simulink library "switchboard"  (R2013a)
settings: Solver=ode3  StartTime=0.0  StopTime=10.0  RelTol=1e-3
libraries: switchboard x2, goto x1
settings Model: Creator=torstebo  LastModifiedBy=torstebo

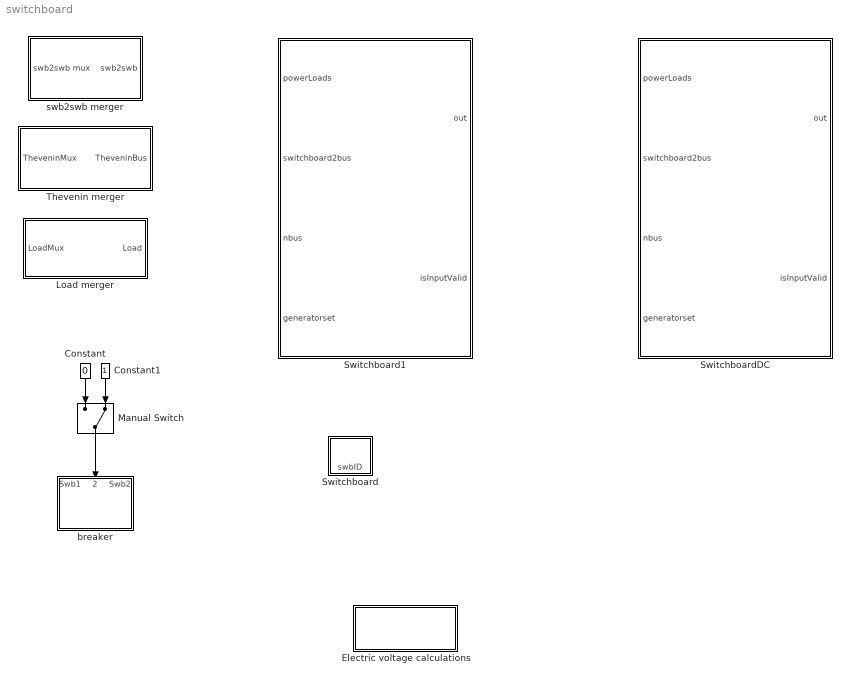
== system switchboard ==
  Constant : Constant  Value=0  OutDataTypeStr=boolean
  Constant1 : Constant  OutDataTypeStr=boolean
  Electric voltage calculations : Subsystem
  Load merger : Subsystem
  Manual Switch : ManualSwitch  CurrentSetting=0
  Switchboard : Subsystem  Tag=Switchboard  mask{swbId=0}
      mask prompts: swbId "Switchboard ID"
  Switchboard1 : MATLAB Function  TreatAsAtomicUnit=on
  SwitchboardDC : MATLAB Function  TreatAsAtomicUnit=on
  Thevenin merger : Subsystem
  breaker : Subsystem  Tag=SwitchboardBreaker  mask{id=0}
  swb2swb merger : Subsystem
  wires:
  Constant/1 -> Manual Switch/1
  Constant1/1 -> Manual Switch/2
  Manual Switch/1 -> breaker/2(Breaker)

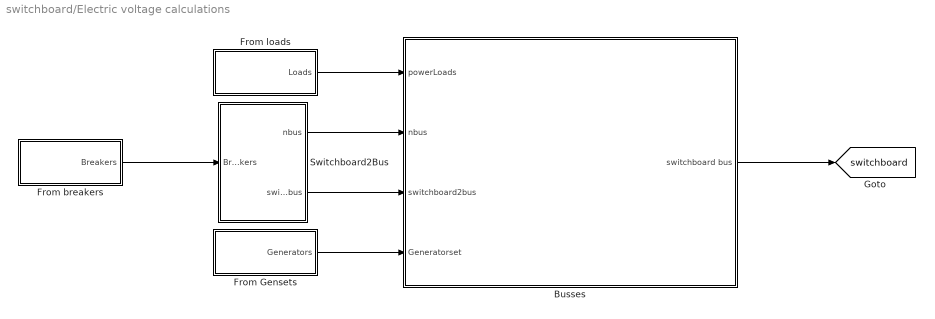
== system switchboard/Electric voltage calculations ==
  Busses : Subsystem
      mask Display:
      | image(imread('figs/switchboard.jpg'))
      | port_label('input',1,'Power Loads')
      | port_label('input',2,'nbus')
      | port_label('input',3,'switchboard2bus')
      | port_label('input',4,'Generators')
      | port_label('output',1,'switchboard')
  From Gensets : Subsystem  Tag=FromGeneratorsetElectric
  From breakers : Subsystem  Tag=FromBreakers
  From loads : Subsystem  Tag=FromLoads
  Switchboard2Bus : Subsystem  Tag=Switchboard2Bus  mask{nSwitchboards=3}
      mask prompts: nSwitchboards "Number of Switchboards"
  tag scope: switchboard=global
  wires:
  From breakers/1(Breakers) -> Switchboard2Bus/1(Breakers)
  From loads/1(Loads) -> Busses/1(powerLoads)
  From Gensets/1(Generators) -> Busses/4(Generatorset)
  Switchboard2Bus/2(switchboard2bus) -> Busses/3(switchboard2bus)
  Switchboard2Bus/1(nbus) -> Busses/2(nbus)
  Busses/1(switchboard bus) -> [switchboard]

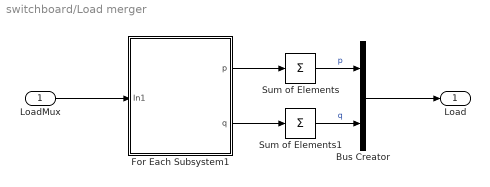
== system switchboard/Load merger ==
  LoadMux : Inport
  Bus Creator : BusCreator  Inputs='p','q'  OutDataTypeStr=Bus: powerLoadsBus  NonVirtualBus=on
  For Each Subsystem1 : Subsystem  TreatAsAtomicUnit=on
  Sum of Elements : Sum  Inputs=+
  Sum of Elements1 : Sum  Inputs=+
  Load : Outport  OutDataTypeStr=Bus: powerLoadsBus
  wires:
  For Each Subsystem1/2(q) -> Sum of Elements1/1
  Sum of Elements1/1 -> Bus Creator/2  "q"
  Sum of Elements/1 -> Bus Creator/1  "p"
  For Each Subsystem1/1(p) -> Sum of Elements/1
  Bus Creator/1 -> Load/1
  LoadMux/1 -> For Each Subsystem1/1(In1)

== system switchboard/Switchboard ==
  Switchboard : Constant  Value=swbId
  swbID : Outport
  wires:
  Switchboard/1 -> swbID/1

== system switchboard/Thevenin merger ==
  TheveninMux : Inport
  For Each Subsystem : Subsystem  TreatAsAtomicUnit=on
  MATLAB Function : MATLAB Function  TreatAsAtomicUnit=on
  TheveninBus : Outport  OutDataTypeStr=Bus: TheveninBus
  wires:
  For Each Subsystem/5(omega) -> MATLAB Function/5(omega)
  For Each Subsystem/2(z) -> MATLAB Function/2(z)
  For Each Subsystem/1(e) -> MATLAB Function/1(e)
  TheveninMux/1 -> For Each Subsystem/1(In1)
  For Each Subsystem/4(Connected) -> MATLAB Function/4(on)
  MATLAB Function/1(thevenin_bus) -> TheveninBus/1
  For Each Subsystem/3(Sb) -> MATLAB Function/3(Sb)

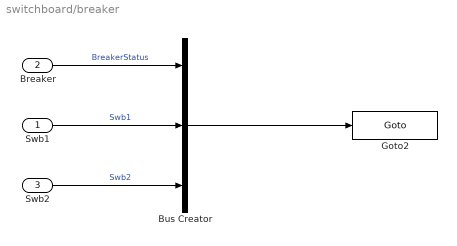
== system switchboard/breaker ==
  Swb1 : Inport
  Breaker : Inport  Port=2
  Swb2 : Inport  Port=3
  Bus Creator : BusCreator  Inputs=3  OutDataTypeStr=Bus: Breaker  NonVirtualBus=on
  Goto2 : goto/Goto  GotoTag=sprintf('Breaker%d',id)
  wires:
  Swb1/1 -> Bus Creator/2  "Swb1"
  Breaker/1 -> Bus Creator/1  "BreakerStatus"
  Swb2/1 -> Bus Creator/3  "Swb2"
  Bus Creator/1 -> Goto2/1

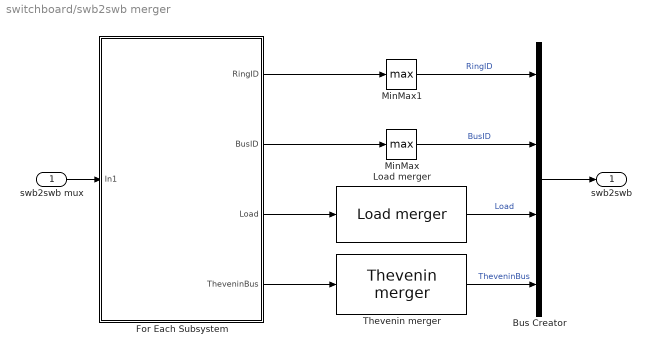
== system switchboard/swb2swb merger ==
  swb2swb mux : Inport
  Bus Creator : BusCreator  Inputs='RingID','BusID','Load','TheveninBus'  OutDataTypeStr=Bus: swb2swb  NonVirtualBus=on
  For Each Subsystem : Subsystem  TreatAsAtomicUnit=on
  Load merger : switchboard/Load merger
  MinMax : MinMax  Function=max
  MinMax1 : MinMax  Function=max
  Thevenin merger : switchboard/Thevenin merger
  swb2swb : Outport  OutDataTypeStr=Bus: swb2swb
  wires:
  For Each Subsystem/1(RingID) -> MinMax1/1
  MinMax1/1 -> Bus Creator/1  "RingID"
  MinMax/1 -> Bus Creator/2  "BusID"
  Thevenin merger/1 -> Bus Creator/4  "TheveninBus"
  Load merger/1 -> Bus Creator/3  "Load"
  For Each Subsystem/2(BusID) -> MinMax/1
  For Each Subsystem/3(Load) -> Load merger/1
  For Each Subsystem/4(TheveninBus) -> Thevenin merger/1
  swb2swb mux/1 -> For Each Subsystem/1(In1)
  Bus Creator/1 -> swb2swb/1

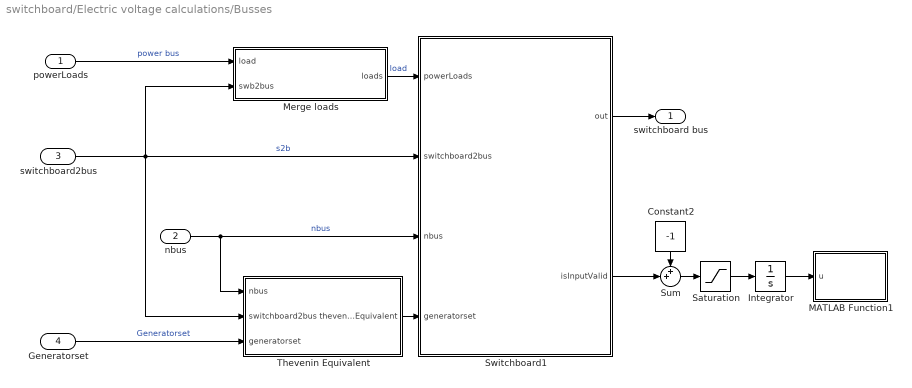
== system switchboard/Electric voltage calculations/Busses ==
  powerLoads : Inport  OutDataTypeStr=Bus: powerLoadsBus
  nbus : Inport  Port=2
  switchboard2bus : Inport  Port=3
  Generatorset : Inport  Port=4
  Constant2 : Constant  Value=-1
  Integrator : Integrator
  MATLAB Function1 : MATLAB Function  TreatAsAtomicUnit=on
  Merge loads : MATLAB Function  TreatAsAtomicUnit=on
  Saturation : Saturate  UpperLimit=0  LowerLimit=-1
  Sum : Sum  Inputs=++|
  Switchboard1 : MATLAB Function  TreatAsAtomicUnit=on
  Thevenin Equivalent : MATLAB Function  TreatAsAtomicUnit=on
  switchboard bus : Outport
  wires:
  Switchboard1/1(out) -> switchboard bus/1
  powerLoads/1 -> Merge loads/1(load)  "power bus"
  switchboard2bus/1 -> Switchboard1/2(switchboard2bus), Merge loads/2(swb2bus), Thevenin Equivalent/2(switchboard2bus)  "s2b"
  Generatorset/1 -> Thevenin Equivalent/3(generatorset)  "Generatorset"
  Integrator/1 -> MATLAB Function1/1(u)
  Constant2/1 -> Sum/1
  Sum/1 -> Saturation/1
  Switchboard1/2(isInputValid) -> Sum/2
  nbus/1 -> Switchboard1/3(nbus), Thevenin Equivalent/1(nbus)  "nbus"
  Merge loads/1(loads) -> Switchboard1/1(powerLoads)  "load"
  Thevenin Equivalent/1(theveninEquivalent) -> Switchboard1/4(generatorset)
  Saturation/1 -> Integrator/1

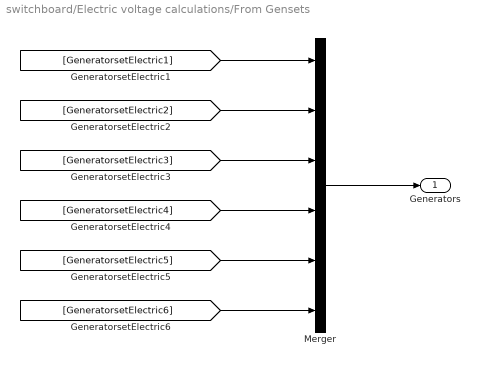
== system switchboard/Electric voltage calculations/From Gensets ==
  Merger : Concatenate  Tag=FromGeneratorsetElectric/Merger  NumInputs=6
  Generators : Outport
  wires:
  Merger/1 -> Generators/1
  [GeneratorsetElectric1] -> Merger/1
  [GeneratorsetElectric2] -> Merger/2
  [GeneratorsetElectric6] -> Merger/6
  [GeneratorsetElectric3] -> Merger/3
  [GeneratorsetElectric4] -> Merger/4
  [GeneratorsetElectric5] -> Merger/5

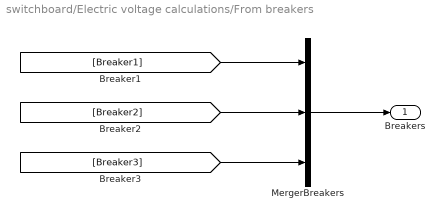
== system switchboard/Electric voltage calculations/From breakers ==
  MergerBreakers : Concatenate  Tag=FromBreakers/MergerBreakers  NumInputs=3
  Breakers : Outport
  wires:
  MergerBreakers/1 -> Breakers/1
  [Breaker1] -> MergerBreakers/1
  [Breaker2] -> MergerBreakers/2
  [Breaker3] -> MergerBreakers/3

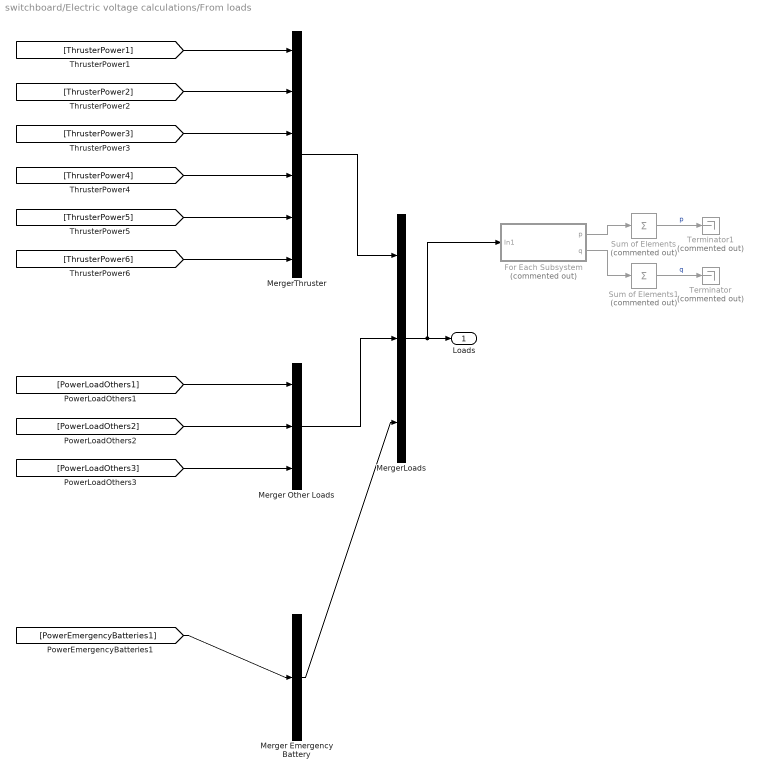
== system switchboard/Electric voltage calculations/From loads ==
  For Each Subsystem : Subsystem  Commented=on  TreatAsAtomicUnit=on
  Merger Emergency Battery : Concatenate  Tag=FromLoads/MergerEmergencyBattery  NumInputs=1
  Merger Other Loads : Concatenate  Tag=FromLoads/MergerOtherLoads  NumInputs=3
  MergerLoads : Concatenate  Tag=FromLoads/MergerLoads  NumInputs=3
  MergerThruster : Concatenate  Tag=FromLoads/MergerThruster  NumInputs=6
  Sum of Elements : Sum  Commented=on  Inputs=+
  Sum of Elements1 : Sum  Commented=on  Inputs=+
  Terminator : Terminator  Commented=on
  Terminator1 : Terminator  Commented=on
  Loads : Outport
  wires:
  MergerThruster/1 -> MergerLoads/1
  Merger Other Loads/1 -> MergerLoads/2
  MergerLoads/1 -> For Each Subsystem/1(In1), Loads/1
  For Each Subsystem/1(p) -> Sum of Elements/1
  For Each Subsystem/2(q) -> Sum of Elements1/1
  Sum of Elements1/1 -> Terminator/1  "q"
  Sum of Elements/1 -> Terminator1/1  "p"
  Merger Emergency Battery/1 -> MergerLoads/3
  [PowerLoadOthers1] -> Merger Other Loads/1
  [PowerLoadOthers2] -> Merger Other Loads/2
  [PowerLoadOthers3] -> Merger Other Loads/3
  [ThrusterPower1] -> MergerThruster/1
  [ThrusterPower2] -> MergerThruster/2
  [ThrusterPower3] -> MergerThruster/3
  [ThrusterPower4] -> MergerThruster/4
  [ThrusterPower5] -> MergerThruster/5
  [ThrusterPower6] -> MergerThruster/6
  [PowerEmergencyBatteries1] -> Merger Emergency Battery/1

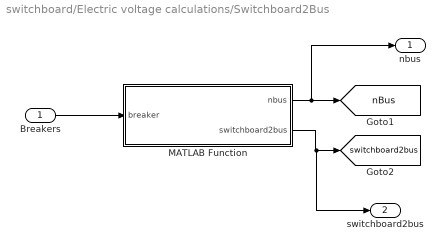
== system switchboard/Electric voltage calculations/Switchboard2Bus ==
  Breakers : Inport
  MATLAB Function : MATLAB Function  TreatAsAtomicUnit=on
  nbus : Outport
  switchboard2bus : Outport  Port=2
  tag scope: nBus=global, switchboard2bus=global
  wires:
  MATLAB Function/2(switchboard2bus) -> switchboard2bus/1, [switchboard2bus]
  MATLAB Function/1(nbus) -> nbus/1, [nBus]
  Breakers/1 -> MATLAB Function/1(breaker)

== system switchboard/Load merger/For Each Subsystem1 ==
  In1 : Inport  OutDataTypeStr=Bus: powerLoadsBus  Partition=on  PartitionDimension=1  PartitionWidth=1
  Bus Selector : BusSelector  OutputSignals=p,q
  For Each : ForEach  DisableCoverage=on  IndexMode=One-based
  p : Outport  ConcatenationDimension=1
  q : Outport  Port=2  ConcatenationDimension=1
  wires:
  Bus Selector/2 -> q/1  "<q>"
  Bus Selector/1 -> p/1  "<p>"
  In1/1 -> Bus Selector/1

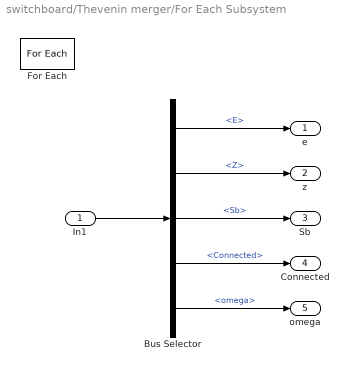
== system switchboard/Thevenin merger/For Each Subsystem ==
  In1 : Inport  OutDataTypeStr=Bus: TheveninBus  Partition=on  PartitionDimension=1  PartitionWidth=1
  Bus Selector : BusSelector  OutputSignals=E,Z,Sb,Connected,omega
  For Each : ForEach  DisableCoverage=on  IndexMode=One-based
  e : Outport  ConcatenationDimension=1
  z : Outport  Port=2  ConcatenationDimension=1
  Sb : Outport  Port=3  ConcatenationDimension=1
  Connected : Outport  Port=4  ConcatenationDimension=1
  omega : Outport  Port=5  ConcatenationDimension=1
  wires:
  Bus Selector/5 -> omega/1  "<omega>"
  In1/1 -> Bus Selector/1
  Bus Selector/1 -> e/1  "<E>"
  Bus Selector/2 -> z/1  "<Z>"
  Bus Selector/3 -> Sb/1  "<Sb>"
  Bus Selector/4 -> Connected/1  "<Connected>"

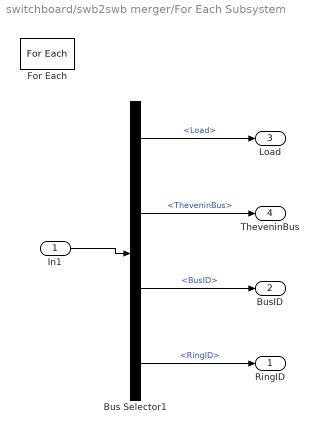
== system switchboard/swb2swb merger/For Each Subsystem ==
  In1 : Inport  OutDataTypeStr=Bus: swb2swb  Partition=on  PartitionDimension=1  PartitionWidth=1
  Bus Selector1 : BusSelector  OutputSignals=Load,TheveninBus,BusID,RingID
  For Each : ForEach  DisableCoverage=on  IndexMode=One-based
  RingID : Outport  OutDataTypeStr=double  ConcatenationDimension=1
  BusID : Outport  Port=2  OutDataTypeStr=uint8  ConcatenationDimension=1
  Load : Outport  Port=3  OutDataTypeStr=Bus: powerLoadsBus  ConcatenationDimension=1
  TheveninBus : Outport  Port=4  OutDataTypeStr=Bus: TheveninBus  ConcatenationDimension=1
  wires:
  Bus Selector1/1 -> Load/1  "<Load>"
  Bus Selector1/4 -> RingID/1  "<RingID>"
  In1/1 -> Bus Selector1/1
  Bus Selector1/3 -> BusID/1  "<BusID>"
  Bus Selector1/2 -> TheveninBus/1  "<TheveninBus>"

== system switchboard/Electric voltage calculations/From loads/For Each Subsystem ==
  In1 : Inport  Partition=on  PartitionDimension=1  PartitionWidth=1
  Bus Selector : BusSelector  OutputSignals=p,q
  For Each : ForEach  DisableCoverage=on  IndexMode=One-based
  p : Outport  ConcatenationDimension=1
  q : Outport  Port=2  ConcatenationDimension=1
  wires:
  In1/1 -> Bus Selector/1
  Bus Selector/1 -> p/1  "<p>"
  Bus Selector/2 -> q/1  "<q>"

== matlab function switchboard/SwitchboardDC ==
  data: powerLoads input; out output Bus: swb; isInputValid output size=1; switchboard2bus input; nbus input; generatorset input
function [out, isInputValid]= switchboardDC(powerLoads,switchboard2bus,nbus,generatorset)
%#codegen

[out, isInputValid]= switchboardCentralDC(powerLoads,switchboard2bus,nbus,generatorset);

== matlab function switchboard/Electric voltage calculations/Busses/MATLAB Function1 ==
  data: u input
function stopper(u)
%#codegen
if ( u < -1)
    error('Bus voltage calculations have been invalid for 1 second, stopping stimulation');
end

== matlab function switchboard/Switchboard1 ==
  data: powerLoads input; out output Bus: swb; isInputValid output size=1; switchboard2bus input; nbus input; generatorset input
function [out, isInputValid]= switchboard(powerLoads,switchboard2bus,nbus,generatorset)
%#codegen

[out, isInputValid]= switchboardCentral(powerLoads,switchboard2bus,nbus,generatorset);

== matlab function switchboard/Electric voltage calculations/Busses/Merge loads ==
  data: load input; loads output Bus: powerLoadsBus; swb2bus input
function loads  = mergeloads(load,swb2bus)
%#codegen
loads = repmat( struct( 'p',0,'q',0,'SwitchboardID',0),length(swb2bus),1);
for i = 1:length(load)
    bus = swb2bus(load(i).SwitchboardID);
    loads(bus).p = loads(bus).p+ load(i).p;
    loads(bus).q = loads(bus).q+ load(i).q;
end
for i = 1:length(swb2bus)
    loads(i).SwitchboardID = i;
end

== matlab function switchboard/Electric voltage calculations/Busses/Switchboard1 ==
  data: powerLoads input; out output Bus: swb; isInputValid output size=1; switchboard2bus input; nbus input; generatorset input
function [out, isInputValid]= switchboard(powerLoads,switchboard2bus,nbus,generatorset)
%#codegen

[out, isInputValid]= switchboardCentral(powerLoads,switchboard2bus,nbus,generatorset);

== matlab function switchboard/Thevenin merger/MATLAB Function ==
  data: e input double; thevenin_bus output Bus: TheveninBus size=1; z input; Sb input; on input; omega input
function thevenin_bus  = TheveninEquivalentWrapper( e, z,Sb, on, omega )%#codegen
%#codegen


[ et, zt, Sb_bus, on, omegaAvg ] = TheveninEquivalent( e, z, Sb, on, omega );

thevenin_bus = struct('E',et,'Z',zt,'Sb',Sb_bus,'Connected',on,'omega',omegaAvg);

== matlab function switchboard/Electric voltage calculations/Switchboard2Bus/MATLAB Function ==
  data: breaker input; nbus output size=1; nSwitchboards parameter size=1; switchboard2bus output size=nSwitchboards
function [nbus, switchboard2bus] = breaker2bus(breaker,nSwitchboards)
%#codegen
    switchboard2bus = (1:nSwitchboards)';
    for i = 1:length(breaker)
        if (breaker(i).BreakerStatus)
            swb1 = breaker(i).Swb1;
            swb2 = breaker(i).Swb2;
            busId1 = switchboard2bus(swb1);
            busId2 = switchboard2bus(swb2);
            busId = min(busId1,busId2);
            switchboard2bus(swb1) = busId;
            switchboard2bus(swb2) = busId;
        end
    end
    
nbus = 0;

for i = 1:nSwitchboards
   if switchboard2bus(i) == i;
       nbus = nbus +1;
       switchboard2bus(i) = nbus;
   else 
       switchboard2bus(i) = switchboard2bus(switchboard2bus(i));
   end
end

end

== matlab function switchboard/Electric voltage calculations/Busses/Thevenin Equivalent ==
  data: nbus input; switchboard2bus input; generatorset input; theveninEquivalent output Bus: TheveninBus
function theveninEquivalent  = mergeGenerators(nbus,switchboard2bus,generatorset)
%#codegen
nSwitchboards = length(switchboard2bus);
assert(nbus<=nSwitchboards);
nGeneratorset = length(generatorset);
E = complex(zeros(nGeneratorset,1));
Z = complex(zeros(nGeneratorset,1));
Sb = zeros(nGeneratorset,1);
Connected = zeros(nGeneratorset,1);
omega = zeros(nGeneratorset,1);
genset2swb = zeros(nGeneratorset,1);
for i = 1:nGeneratorset
    E(i) = generatorset(i).E;
    Z(i) = generatorset(i).Z;
    Sb(i) = generatorset(i).Sb;
    Connected(i) = generatorset(i).Connected;
    omega(i) = generatorset(i).omega;
    genset2swb(i) = generatorset(i).SwitchboardID;
end   

theveninEquivalent = repmat( struct( 'E',1j,'Z',1j,'Sb',0,'Connected',true,'omega',0,'SwitchboardID',0),nSwitchboards);
for bus = 1:nbus
    %Find gensets connected to bus
    m = 0;  
    for i = 1:nGeneratorset
        if (switchboard2bus(genset2swb(i))==bus && Connected(i))
            m = m + 1;
        end
    end
    assert(m <= nGeneratorset);
    gensets = zeros(1,m);
    m = 0;    
    for i = 1:nGeneratorset
        if (switchboard2bus(genset2swb(i))==bus && Connected(i))
            m = m + 1;
            gensets(m) = i;
        end
    end
    [ et, zt, Sb_bus, ~, omegaAvgBus ] = TheveninEquivalent( E(gensets), Z(gensets), Sb(gensets), Connected(gensets), omega(gensets) );
    theveninEquivalent(bus).E = et;
    theveninEquivalent(bus).Z = zt;
    theveninEquivalent(bus).Sb = Sb_bus;
    theveninEquivalent(bus).Connected = true;
    theveninEquivalent(bus).omega = omegaAvgBus;
    theveninEquivalent(bus).SwitchboardID = bus;
end
